simulink subsystem "pendulum"  (R2025b)
settings: Solver=VariableStepAuto  StartTime=0.0  StopTime=10.0  RelTol=1e-3
model mask{y0=0.1, dy0=0, u0=0}
  mask prompts: y0 "Initial Angular Position"; dy0 "Initial Angular velocity"; u0 "Initial Control Force"
settings Model: Creator=brianli  LastModifiedBy=brianli

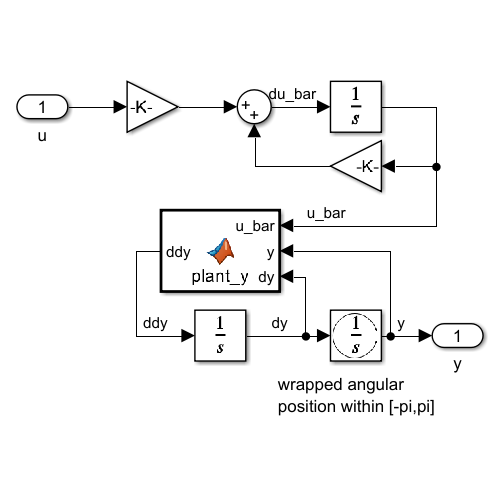
[thumbnail: Simulink's stored preview of the top-level diagram]
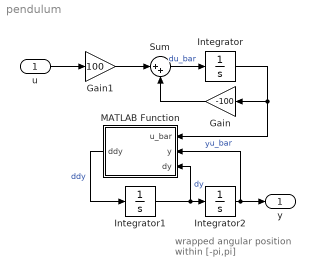
== system pendulum ==
  note: wrapped angular
      | position within [-pi,pi]
  u : Inport
  Gain : Gain  Gain=-100
  Gain1 : Gain  Gain=100
  Integrator : Integrator  InitialCondition=u0
  Integrator1 : Integrator  InitialCondition=dy0
  Integrator2 : Integrator  InitialCondition=y0  WrapState=on  ZeroCross=off
  MATLAB Function : MATLAB Function  TreatAsAtomicUnit=on
  Sum : Sum  Inputs=|++
  y : Outport
  wires:
  u/1 -> Gain1/1
  Integrator1/1 -> MATLAB Function/3(dy), Integrator2/1  "dy"
  Integrator/1 -> Gain/1, MATLAB Function/1(u_bar)  "u_bar"
  Gain1/1 -> Sum/1
  Gain/1 -> Sum/2
  Sum/1 -> Integrator/1  "du_bar"
  MATLAB Function/1(ddy) -> Integrator1/1  "ddy"
  Integrator2/1 -> y/1, MATLAB Function/2(y)  "y"

== matlab function pendulum/MATLAB Function ==
  data: u_bar input; ddy output; y input; dy input
function ddy = plant_y(u_bar,y,dy)

num = 9.8*sin(y) + cos(y) * (-u_bar - 0.25 * dy^2 * sin(y)) / 1.5;
den = 0.5 * (4/3 - 1/3 * cos(y)^2);

ddy = num/den;
